simulink model "MMC"  (Simulink 10.0)
settings: Solver=ode45  StartTime=0.0  StopTime=0.08  MaxStep=1e-6  RelTol=1e-3  EnableMultiTasking=on
libraries: powerlib x12, simulink x4
settings Model: Creator=Administrator  LastModifiedBy=29721
settings DataIOCC: LimitDataPoints=on  SignalLoggingSaveFormat=ModelDataLogs
settings OptimizationCC: ExpressionDepthLimit=2147483647
settings DebuggingCC: SolverPrmCheckMsg=warning  FcnCallInpInsideContextMsg=warning  StateNameClashWarn=warning
settings GRTTargetCC: GeneratePreprocessorConditionals=Disable all  CombineOutputUpdateFcns=on  GRTInterface=off
settings ConfigComp: CovExternalEMLEnable=off  CovSFcnEnable=off
settings SimscapeCC: SimscapeNormalizeSystem=off

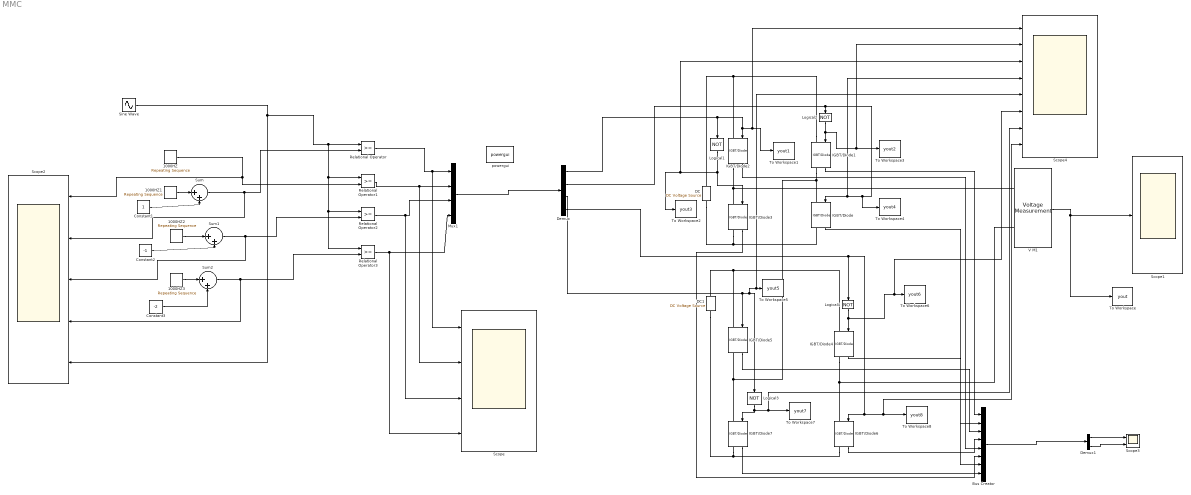
== system MMC ==
  1000HZ{,1..3} (4 alike) : simulink/Sources/Repeating Sequence  rep_seq_t=[0 1/4000 2/4000 4/4000]  rep_seq_y=[0 0.5 1 0]
  Bus Creator : BusCreator  Inputs=8
  Constant1 : Constant
  Constant2 : Constant  Value=-1
  Constant3 : Constant  Value=-2
  DC : powerlib/Electrical Sources/DC Voltage Source  Amplitude=100  Measurements=None
      settings: SourceProductName=Simscape Electrical
  DC1 : powerlib/Electrical Sources/DC Voltage Source  Amplitude=100  Measurements=None
      settings: SourceProductName=Simscape Electrical
  Demux : Demux
  Demux1 : Demux  Outputs=2
  IGBT/Diode{,1..7} (8 alike) : powerlib/Power Electronics/IGBT//Diode  Ron=1e-3  Rs=1e5  Cs=inf  Measurements=on
      settings: SourceProductName=Simscape Electrical
  Logical{1..4} (4 alike) : Logic  Operator=NOT  AllPortsSameDT=off  OutDataTypeStr=boolean
  Mux1 : Mux
  Relational Operator{,1..3} (4 alike) : RelationalOperator  OutDataTypeStr=boolean  RndMeth=Nearest
  Scope : Scope  NumInputPorts=4
  Scope1 : Scope
  Scope2 : Scope  NumInputPorts=5
  Scope3 : Scope  NumInputPorts=2
  Scope4 : Scope  NumInputPorts=8
  Sine Wave : Sin  Amplitude=1.6  Frequency=314  SampleTime=0
  Sum : Sum  Inputs=|++
  Sum1 : Sum  Inputs=|++
  Sum2 : Sum  Inputs=|++
  To Workspace : ToWorkspace  VariableName=yout  SampleTime=-1
      settings: Save2DSignal=2-D array (concatenate along first dimension)
  To Workspace1 : ToWorkspace  VariableName=yout1  SampleTime=-1
      settings: Save2DSignal=2-D array (concatenate along first dimension)
  To Workspace2 : ToWorkspace  VariableName=yout3  SampleTime=-1
      settings: Save2DSignal=2-D array (concatenate along first dimension)
  To Workspace3 : ToWorkspace  VariableName=yout2  SampleTime=-1
      settings: Save2DSignal=2-D array (concatenate along first dimension)
  To Workspace4 : ToWorkspace  VariableName=yout4  SampleTime=-1
      settings: Save2DSignal=2-D array (concatenate along first dimension)
  To Workspace5 : ToWorkspace  VariableName=yout5  SampleTime=-1
      settings: Save2DSignal=2-D array (concatenate along first dimension)
  To Workspace6 : ToWorkspace  VariableName=yout6  SampleTime=-1
      settings: Save2DSignal=2-D array (concatenate along first dimension)
  To Workspace7 : ToWorkspace  VariableName=yout7  SampleTime=-1
      settings: Save2DSignal=2-D array (concatenate along first dimension)
  To Workspace8 : ToWorkspace  VariableName=yout8  SampleTime=-1
      settings: Save2DSignal=2-D array (concatenate along first dimension)
  V M1 : powerlib/Measurements/Voltage Measurement  PhasorSimulation=off  OutputType=Complex  PSBequivalent=0
      settings: SourceProductName=Simscape Electrical
  powergui : powerlib/powergui  Priority=1  SimulationMode=Discrete  SampleTime=40e-6  frequency=60  Iterations=50  frequencyindice=0  Pbase=100e6  ErrMax=1e-4  UnitsV=kV  UnitsW=MW  buscounter=0  FunctionMessages=off  echomessages=off  EnableUseOfTLC=off  CurrentSourceSwitches=off  DisableSnubberDevices=off  DisableRonSwitches=off  DisableVfSwitches=off  DisplayEquations=off  AutomaticDiscreteSolvers=off  SolverType=Tustin  Interpol=off  ExternalGateDelay=off  methode=off  Ts=0  x0status=blocks  SPID=off  SwTol=0  HookPort=off  NonlinearTolerance=1e-4  nMaxIteration=100  ContinueOnMaxIteration=off  RestoreLinks=warning  ResistiveCurrentMeasurement=off  Frange=[0:2:500]  Ylog=off  Xlog=on  ShowGrid=off  save=off  variable=ZData  structure=yout  ZoomFFT=off  StartTime=0  cycles=2  DisplayStyle=1  fundamental=50  FreqAxis=off  MaxFrequency=1000  frequencyindicesteady=1  RmsSteady=1  display=off
      settings: SourceProductName=Simscape Electrical
  wires:
  Demux/2 -> To Workspace4/1, Scope4/4, IGBT/Diode/1, Logical2/1
  Logical3/1 -> Scope4/7, To Workspace7/1, IGBT/Diode7/1
  Demux/3 -> IGBT/Diode5/1, Scope4/5, To Workspace5/1, Logical3/1
  Logical2/1 -> Scope4/2, To Workspace3/1, IGBT/Diode1/1
  Demux/4 -> Scope4/8, To Workspace8/1, IGBT/Diode6/1, Logical4/1
  Logical1/1 -> Scope4/3, To Workspace2/1, IGBT/Diode3/1
  Demux/1 -> Scope4/1, To Workspace1/1, IGBT/Diode2/1, Logical1/1
  1000HZ/1 -> Relational Operator1/2, Scope2/1
  Relational Operator1/1 -> Scope/2, Mux1/2
  Sine Wave/1 -> Scope2/5, Relational Operator1/1, Relational Operator2/1, Relational Operator3/1, Relational Operator/1
  Mux1/1 -> Demux/1
  Relational Operator/1 -> Scope/1, Mux1/1
  Relational Operator2/1 -> Scope/3, Mux1/3
  Relational Operator3/1 -> Scope/4, Mux1/4
  Sum/1 -> Scope2/2, Relational Operator/2
  Sum1/1 -> Scope2/3, Relational Operator2/2
  Sum2/1 -> Scope2/4, Relational Operator3/2
  1000HZ1/1 -> Sum/1
  Constant1/1 -> Sum/2
  1000HZ2/1 -> Sum1/1
  Constant2/1 -> Sum1/2
  1000HZ3/1 -> Sum2/1
  Constant3/1 -> Sum2/2
  V M1/1 -> To Workspace/1, Scope1/1
  Demux1/1 -> Scope3/1
  Demux1/2 -> Scope3/2
  IGBT/Diode/1 -> Bus Creator/7
  IGBT/Diode1/1 -> Bus Creator/1
  Bus Creator/1 -> Demux1/1
  IGBT/Diode2/1 -> Bus Creator/5
  IGBT/Diode3/1 -> Bus Creator/6
  IGBT/Diode4/1 -> Bus Creator/2
  IGBT/Diode5/1 -> Bus Creator/3
  IGBT/Diode6/1 -> Bus Creator/4
  IGBT/Diode7/1 -> Bus Creator/8
  Logical4/1 -> Scope4/6, To Workspace6/1, IGBT/Diode4/1
  connections:
  DC1/LConn1 -- IGBT/Diode7/RConn1 -- IGBT/Diode6/RConn1
  DC/LConn1 -- IGBT/Diode/RConn1 -- IGBT/Diode3/RConn1
  IGBT/Diode7/LConn1 -- IGBT/Diode5/RConn1 -- IGBT/Diode/LConn1 -- IGBT/Diode1/RConn1
  DC1/RConn1 -- IGBT/Diode4/LConn1 -- IGBT/Diode5/LConn1
  V M1/LConn2 -- IGBT/Diode6/LConn1 -- IGBT/Diode4/RConn1
  IGBT/Diode1/LConn1 -- IGBT/Diode2/LConn1 -- DC/RConn1
  V M1/LConn1 -- IGBT/Diode2/RConn1 -- IGBT/Diode3/LConn1
